simulink model "SF5_5_14_jc0491"  (R2016b)
settings: Solver=VariableStepAuto  StartTime=0.0  StopTime=10.0  RelTol=1e-3  EnableMultiTasking=on
settings Model: Creator=amyyang  LastModifiedBy=amyyang
settings DataIOCC: LimitDataPoints=on
settings OptimizationCC: LifeSpan=inf
settings DebuggingCC: AllowSymbolicDim=off  SFUnexpectedBacktrackingDiag=warning  SFNoUnconditionalDefaultTransitionDiag=warning  SFExecutionAtInitializationDiag=none
settings ModelReferenceCC: PropagateSignalLabelsOutOfModel=off
settings GRTTargetCC: TargetLangStandard=C89/C90 (ANSI)
settings ConfigComp: CovMetricSettings=dw  CovHtmlReporting=on  CovSaveCumulativeToWorkspaceVar=on  CovSaveSingleToWorkspaceVar=on  CovExternalEMLEnable=off

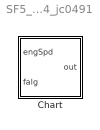
== system SF5_5_14_jc0491 ==
  Chart : Stateflow chart  TreatAsAtomicUnit=on

== stateflow chart SF5_5_14_jc0491/Chart ==
  state A [parallel]
    settings: executionOrder=1
    note: 作为循环计数器的变量，在同一个状态内，就只做这一个用。
    (default) -> (junction 2) : {
        |  i = 1;
        | }
    (junction 2) -> (junction 36) [order 1] : [ i<10]
    (junction 36) -> (junction 38)
    (junction 38) -> (junction 2) : {
        |  i++;
        | }
    (junction 2) -> (junction 40) [order 2] : {
        | c = b + a;
        | }
  state A1 [parallel]
    settings: executionOrder=3
    note: 作为循环计数器的变量，在同一个状态内，就只做这一个用途。
    (default) -> (junction 85) : {
        |  i = 1;
        | }
    (junction 85) -> (junction 87) [order 1] : [ i<10]
    (junction 87) -> (junction 82)
    (junction 82) -> (junction 85) : {
        |  i++;
        | }
    (junction 85) -> (junction 83) [order 2] : {
        | i = b + a;
        | }
  state B [parallel]
    settings: executionOrder=2
    state SA1
      en:
      pre1 = 0;
      pre2 = 0;
      du:
      a = alp * Tin ;
      out = alp*a;
    state SA2
      en:
      a = pre2 - pre1;
      out = Tin*a;
    note: 这里的 a 作为各个state定义的Lcoal变量，需要在各自的state里单独定义
    (default) -> SA1
    SA1 -> SA2 : [ (engSpd < 10) || (engSpd > 9000)]
    SA2 -> SA1 : [ falg ]
  data: i local double; b local double; a local double; c local double; i local double; b local double; a local double; c local double; a local double; a local double; Tin local double; alp local double; pre1 local double; pre2 local double; out output double; engSpd input; falg input
